simulink model "adaptive_observer_for_sin_signal_original"  (R2021b)
settings: Solver=ode4  StartTime=0.0  StopTime=simulationTime  FixedStep=0.0001  RelTol=1e-3
model workspace: external: MATLAB File D:\practice\sci\variables2n1.m (data not in the file)
values from neighbouring files (symbols this model uses):
  A = zeros(2*dimension+1 , 2*dimension+1)    [LCAD.m]
  alpha = [1,3]    [variables2n1.m]
  amp = [1;1]    [variables2n1.m]
  amp_M = [1;1]    [variables2n1.m]
  amp_M1 = 0.2    [variables2n1.m]
  bias = [0;0]    [variables2n1.m]
  bias_M = [0;0]    [variables2n1.m]
  bias_M1 = 0    [variables2n1.m]
  bigGammaZ0 = zeros(2*dimension+1, dimension)    [variables2n1.m]
  C = zeros(1, 2*dimension+1)    [LCAD.m]
  delta = C*A    [LCAD.m]    (also in stats.m = 0.05)
  dimension = 2    [variables2n1.m]
  freq = [2;3]    [variables2n1.m]
  freq_M = [1.8;3.2]    [variables2n1.m]
  freq_M1 = 20    [variables2n1.m]
  freqSwitcher = [80,150]    [variables2n1.m]
  gamma_my = 0.01    [starter3.m]
  h_my = 0.3    [starter3.m]
  initialTheta = [initialOmega(1)^2-alpha(1);     initialOmega(2)^2-alpha(2)]    [variables2n1.m]
  initialZ = [sin(phase(1)); r^2*cos(phase(1))/initialOmega(1);     sin(phase(2)); r^2*cos(phase(2))/initialOmega(2); sum(bias)]    [variables2n1.m]
  k_my = 100    [starter3.m]
  L = real((place(A',C',eigenvalues))')    [LCAD.m]
  mu = 25    [graphs.m]    (also in plot_pres4.m = 2.5; variables2n1.m = 2.5)
  noiseOrSin = 0    [variables2n1.m]
  noiseOrSwitch = 0    [variables2n1.m]
  omega1 = ones(1, length(time))*2    [graphs.m]    (also in starter3.m = 2)
  omega2 = ones(1, length(time))*3    [graphs.m]    (also in starter3.m = 3)
  omega_max = 10    [starter3.m]
  omega_min = 1    [starter3.m]
  omegaLimiter = sqrt(dimension)*maxOmega    [variables2n1.m]
  phase = [0;0]    [variables2n1.m]
  phase_M = [0;0]    [variables2n1.m]
  phase_M1 = 0    [variables2n1.m]
  r = 1.2    [variables2n1.m]
  sample_M1 = 10    [variables2n1.m]
  tau_my = 0.3    [starter3.m]
  theta0_my = [-2; 1]    [starter3.m]
  theta_real = [-c1-c2; c1*c2]    [starter3.m]
  turn_mods_on = 1    [variables2n1.m]
  zMax = 5    [variables2n1.m]
undefined symbols (not defined in the file or in its folder): G, isComplex, L1
libraries: simulink x1
(part 1 of 3)
settings Model: Creator=ASUS  LastModifiedBy=ASUS

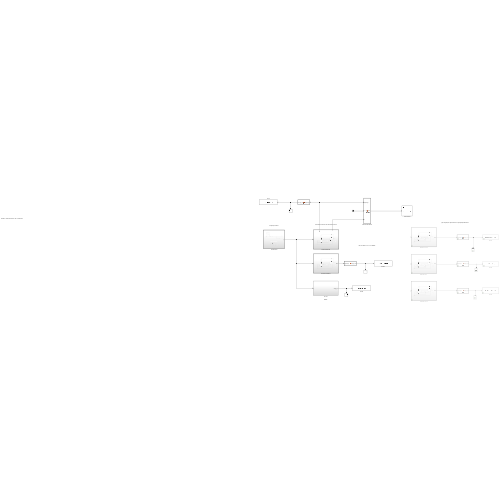
[thumbnail: Simulink's stored preview of the top-level diagram]
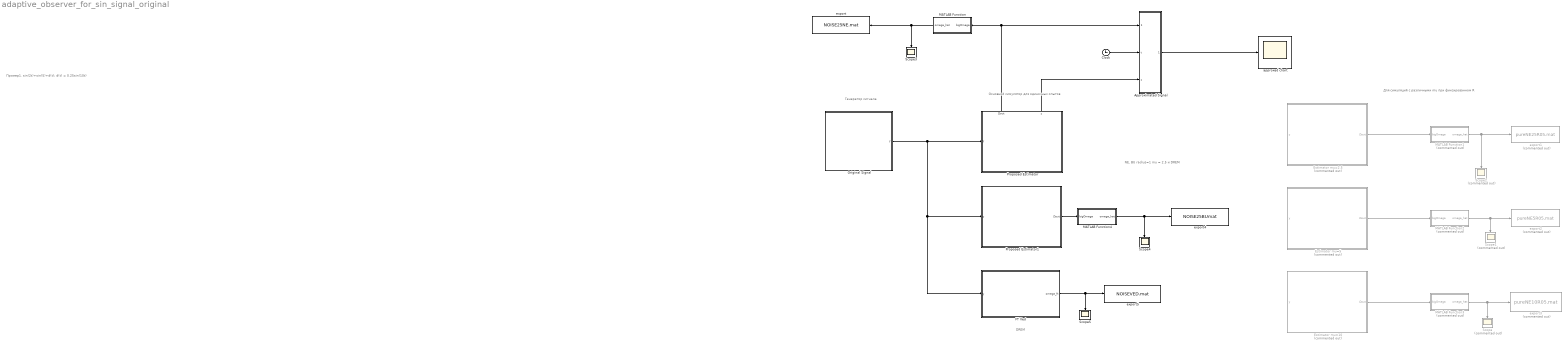
== system adaptive_observer_for_sin_signal_original ==
  note: DREM
  note: Генератор сигнала
  note: Основной симулятор для одиночных опытов
  note: Для симуляций с различными mu при фиксированном R
  note: NE, BU radius=1 mu = 2.5 и DREM
  note: Пример1. sin(2t)+sin(5)+d(t); d(t) = 0.25sin(10t)
  Approximated Signal : MATLAB Function  TreatAsAtomicUnit=on
  Clock : Clock
  Estimator mu=10 : Subsystem  Priority=2  Commented=on  TreatAsAtomicUnit=on
  Estimator mu=2.5 : Subsystem  Priority=2  Commented=on  TreatAsAtomicUnit=on
  Estimator mu=5 : Subsystem  Priority=2  Commented=on  TreatAsAtomicUnit=on
  FT Ved : Subsystem
  MATLAB Function : MATLAB Function  TreatAsAtomicUnit=on
  MATLAB Function1 : MATLAB Function  Commented=on  TreatAsAtomicUnit=on
  MATLAB Function2 : MATLAB Function  Commented=on  TreatAsAtomicUnit=on
  MATLAB Function3 : MATLAB Function  Commented=on  TreatAsAtomicUnit=on
  MATLAB Function4 : MATLAB Function  TreatAsAtomicUnit=on
  Original Signal : Subsystem  Priority=1  TreatAsAtomicUnit=on
  Proposed Estimator : Subsystem  Priority=2  TreatAsAtomicUnit=on
      settings: PortSchema="{\"entries\":[{\"content\":{\"sides\":[{\"content\":{\"connectorIds\":[\"In1\"]},\"type\":\"ConnectorPlacement.EquallySpacedRectSide\",\"uuid\":\"aaf14987-3f40-4b34-b366-ded74c88fbf6\"},{\"content\":{\"connectorIds\":[],\"side\":\"RIGHT\"},\"type\":\"ConnectorPlacement.EquallySpacedRectSide\",\"uuid\":\"c64b6003-6675-4c3e-855a-6bb89f1643de\"},{\"content\":{\"connectorIds\":[\"Out1\",\"Out2\"],\"side\":\"TOP\"},\"type\":\"ConnectorPlacement.EquallySpacedRectSide\",\"uuid\":\"73f281aa-621e-4d37-ab39-3b87d797de55\"}]},\"type\":\"ConnectorPlacement.EquallySpacedConnector\",\"uuid\":\"834767e8-0f9a-475e-a3b3-531c69e18da1\"}],\"packageUris\":[\"http://schema.mathworks.com/mf0/Connector/R2020b\"],\"version\":\"1.0\"}"
  Proposed Estimator1 : Subsystem  Priority=2  TreatAsAtomicUnit=on
  Scope : Scope  Commented=on
  Scope1 : Scope  Commented=on
  Scope2 : Scope  Commented=on
  Scope3 : Scope
  Scope4 : Scope
  Scope5 : Scope
  approxed chart : Scope
  export : ToFile  Filename=NOISE25NE.mat  MatrixName=approx_mu1
  export1 : ToFile  Commented=on  Filename=pureNE25R05.mat  MatrixName=approx_mu2_5
  export2 : ToFile  Commented=on  Filename=pureNE5R05.mat  MatrixName=approx_mu_5
  export3 : ToFile  Commented=on  Filename=pureNE10R05.mat  MatrixName=approx_mu_10
  export4 : ToFile  Filename=NOISE25BUmat  MatrixName=approx_mu1
  export5 : ToFile  Filename=NOISEVED.mat  MatrixName=approx_mu1
  wires:
  Approximated Signal/1(sgn_value) -> approxed chart/1
  Clock/1 -> Approximated Signal/2(t)
  Original Signal/1(y) -> FT Ved/1(y), Proposed Estimator1/1(y), Proposed Estimator/1(y)
  Proposed Estimator/2(z) -> Approximated Signal/3(z)
  Proposed Estimator/1(Ωout) -> Approximated Signal/1(bigOmega), MATLAB Function/1(bigOmega)
  MATLAB Function/1(omega_hat) -> export/1, Scope3/1
  MATLAB Function1/1(omega_hat) -> export1/1, Scope2/1
  Estimator mu=2.5/1(Ωout) -> MATLAB Function1/1(bigOmega)
  Estimator mu=5/1(Ωout) -> MATLAB Function2/1(bigOmega)
  MATLAB Function2/1(omega_hat) -> Scope1/1, export2/1
  Estimator mu=10/1(Ωout) -> MATLAB Function3/1(bigOmega)
  MATLAB Function3/1(omega_hat) -> export3/1, Scope/1
  Proposed Estimator1/1(Ωout) -> MATLAB Function4/1(bigOmega)
  FT Ved/1(omega_ft) -> Scope5/1, export5/1
  MATLAB Function4/1(omega_hat) -> Scope4/1, export4/1

== system adaptive_observer_for_sin_signal_original/Estimator mu=10 ==
  note: Оценщик Ω
  note: Оценщик Φ
  note: Оценщик z
  y : Inport
  Frequencies estimator : Subsystem
      settings: PortSchema="{\"entries\":[{\"content\":{\"sides\":[{\"content\":{\"connectorIds\":[\"In1\",\"In2\"]},\"type\":\"ConnectorPlacement.EquallySpacedRectSide\",\"uuid\":\"56415c13-d553-4f88-94d3-75bcdc800e4b\"},{\"content\":{\"connectorIds\":[\"Out1\"],\"side\":\"RIGHT\"},\"type\":\"ConnectorPlacement.EquallySpacedRectSide\",\"uuid\":\"a1bdd2d2-4e49-40cb-b0b7-1df5316e4510\"},{\"content\":{\"connectorIds\":[\"In3\"],\"side\":\"TOP\"},\"type\":\"ConnectorPlacement.EquallySpacedRectSide\",\"uuid\":\"59b6ba3d-4a55-43e8-9b14-0d873cc3c9ca\"},{\"content\":{\"connectorIds\":[\"In4\",\"In5\"],\"side\":\"BOTTOM\"},\"type\":\"ConnectorPlacement.EquallySpacedRectSide\",\"uuid\":\"70a04625-4f15-4458-8acb-2ccaa963f28c\"}]},\"type\":\"ConnectorPlacement.EquallySpacedConnector\",\"uuid\":\"fdf2e112-ecff-41aa-a5cb-d527a9dd51a8\"}],\"packageUris\":[\"http://schema.mathworks.com/mf0/Connector/R2020b\"],\"version\":\"1.0\"}"
  Subsystem : Subsystem  Priority=6  TreatAsAtomicUnit=on
  Subsystem1 : Subsystem  Commented=on
  z' : Subsystem  Priority=7  TreatAsAtomicUnit=on
      settings: PortSchema="{\"entries\":[{\"content\":{\"sides\":[{\"content\":{\"connectorIds\":[\"In1\",\"In2\"]},\"type\":\"ConnectorPlacement.EquallySpacedRectSide\",\"uuid\":\"ef8cffdc-1e6f-42c0-8cb3-bf318ca182f8\"},{\"content\":{\"connectorIds\":[\"Out1\"],\"side\":\"RIGHT\"},\"type\":\"ConnectorPlacement.EquallySpacedRectSide\",\"uuid\":\"a9c7e5b7-281a-47aa-808a-eb2877f3eee0\"},{\"content\":{\"connectorIds\":[\"In3\"],\"side\":\"TOP\"},\"type\":\"ConnectorPlacement.EquallySpacedRectSide\",\"uuid\":\"7bb4f6b5-7deb-4e08-9b2d-b96cfbb2c85e\"},{\"content\":{\"connectorIds\":[\"In4\"],\"side\":\"BOTTOM\"},\"type\":\"ConnectorPlacement.EquallySpacedRectSide\",\"uuid\":\"fa3b2d15-5a15-4cf8-893e-51642802107c\"}]},\"type\":\"ConnectorPlacement.EquallySpacedConnector\",\"uuid\":\"64fccc24-315d-40ff-920f-bd434d551c1a\"}],\"packageUris\":[\"http://schema.mathworks.com/mf0/Connector/R2020b\"],\"version\":\"1.0\"}"
  Г(z) : MATLAB Function  Priority=2  TreatAsAtomicUnit=on
  "∫Z " : Integrator  Priority=1  InitialCondition=initialZ
  Ωout : Outport
  wires:
  z'/1(z') -> "∫Z "/1, Frequencies estimator/2(ż)
  Г(z)/1(bigGammaZ) -> z'/2(Г(z))
  Frequencies estimator/1(Ω out) -> Subsystem/1(Ω), Frequencies estimator/3(Ω in), Ωout/1
  y/1 -> Frequencies estimator/5(y), z'/1(y)
  Subsystem/1(Ф) -> z'/3(Ф), Frequencies estimator/1(Ф)
  "∫Z "/1 -> Frequencies estimator/4(z), Г(z)/1(z), z'/4(z)

== system adaptive_observer_for_sin_signal_original/Estimator mu=2.5 ==
  note: Оценщик Ω
  note: Оценщик Φ
  note: Оценщик z
  y : Inport
  Frequencies estimator : Subsystem
      settings: PortSchema="{\"entries\":[{\"content\":{\"sides\":[{\"content\":{\"connectorIds\":[\"In1\",\"In2\"]},\"type\":\"ConnectorPlacement.EquallySpacedRectSide\",\"uuid\":\"56415c13-d553-4f88-94d3-75bcdc800e4b\"},{\"content\":{\"connectorIds\":[\"Out1\"],\"side\":\"RIGHT\"},\"type\":\"ConnectorPlacement.EquallySpacedRectSide\",\"uuid\":\"a1bdd2d2-4e49-40cb-b0b7-1df5316e4510\"},{\"content\":{\"connectorIds\":[\"In3\"],\"side\":\"TOP\"},\"type\":\"ConnectorPlacement.EquallySpacedRectSide\",\"uuid\":\"59b6ba3d-4a55-43e8-9b14-0d873cc3c9ca\"},{\"content\":{\"connectorIds\":[\"In4\",\"In5\"],\"side\":\"BOTTOM\"},\"type\":\"ConnectorPlacement.EquallySpacedRectSide\",\"uuid\":\"70a04625-4f15-4458-8acb-2ccaa963f28c\"}]},\"type\":\"ConnectorPlacement.EquallySpacedConnector\",\"uuid\":\"fdf2e112-ecff-41aa-a5cb-d527a9dd51a8\"}],\"packageUris\":[\"http://schema.mathworks.com/mf0/Connector/R2020b\"],\"version\":\"1.0\"}"
  Subsystem : Subsystem  Priority=6  TreatAsAtomicUnit=on
  Subsystem1 : Subsystem  Commented=on
  z' : Subsystem  Priority=7  TreatAsAtomicUnit=on
      settings: PortSchema="{\"entries\":[{\"content\":{\"sides\":[{\"content\":{\"connectorIds\":[\"In1\",\"In2\"]},\"type\":\"ConnectorPlacement.EquallySpacedRectSide\",\"uuid\":\"ef8cffdc-1e6f-42c0-8cb3-bf318ca182f8\"},{\"content\":{\"connectorIds\":[\"Out1\"],\"side\":\"RIGHT\"},\"type\":\"ConnectorPlacement.EquallySpacedRectSide\",\"uuid\":\"a9c7e5b7-281a-47aa-808a-eb2877f3eee0\"},{\"content\":{\"connectorIds\":[\"In3\"],\"side\":\"TOP\"},\"type\":\"ConnectorPlacement.EquallySpacedRectSide\",\"uuid\":\"7bb4f6b5-7deb-4e08-9b2d-b96cfbb2c85e\"},{\"content\":{\"connectorIds\":[\"In4\"],\"side\":\"BOTTOM\"},\"type\":\"ConnectorPlacement.EquallySpacedRectSide\",\"uuid\":\"fa3b2d15-5a15-4cf8-893e-51642802107c\"}]},\"type\":\"ConnectorPlacement.EquallySpacedConnector\",\"uuid\":\"64fccc24-315d-40ff-920f-bd434d551c1a\"}],\"packageUris\":[\"http://schema.mathworks.com/mf0/Connector/R2020b\"],\"version\":\"1.0\"}"
  Г(z) : MATLAB Function  Priority=2  TreatAsAtomicUnit=on
  "∫Z " : Integrator  Priority=1  InitialCondition=initialZ
  Ωout : Outport
  wires:
  z'/1(z') -> "∫Z "/1, Frequencies estimator/2(ż)
  Г(z)/1(bigGammaZ) -> z'/2(Г(z))
  Frequencies estimator/1(Ω out) -> Subsystem/1(Ω), Frequencies estimator/3(Ω in), Ωout/1
  y/1 -> Frequencies estimator/5(y), z'/1(y)
  Subsystem/1(Ф) -> z'/3(Ф), Frequencies estimator/1(Ф)
  "∫Z "/1 -> Frequencies estimator/4(z), Г(z)/1(z), z'/4(z)

== system adaptive_observer_for_sin_signal_original/Estimator mu=5 ==
  note: Оценщик Ω
  note: Оценщик Φ
  note: Оценщик z
  y : Inport
  Frequencies estimator : Subsystem
      settings: PortSchema="{\"entries\":[{\"content\":{\"sides\":[{\"content\":{\"connectorIds\":[\"In1\",\"In2\"]},\"type\":\"ConnectorPlacement.EquallySpacedRectSide\",\"uuid\":\"56415c13-d553-4f88-94d3-75bcdc800e4b\"},{\"content\":{\"connectorIds\":[\"Out1\"],\"side\":\"RIGHT\"},\"type\":\"ConnectorPlacement.EquallySpacedRectSide\",\"uuid\":\"a1bdd2d2-4e49-40cb-b0b7-1df5316e4510\"},{\"content\":{\"connectorIds\":[\"In3\"],\"side\":\"TOP\"},\"type\":\"ConnectorPlacement.EquallySpacedRectSide\",\"uuid\":\"59b6ba3d-4a55-43e8-9b14-0d873cc3c9ca\"},{\"content\":{\"connectorIds\":[\"In4\",\"In5\"],\"side\":\"BOTTOM\"},\"type\":\"ConnectorPlacement.EquallySpacedRectSide\",\"uuid\":\"70a04625-4f15-4458-8acb-2ccaa963f28c\"}]},\"type\":\"ConnectorPlacement.EquallySpacedConnector\",\"uuid\":\"fdf2e112-ecff-41aa-a5cb-d527a9dd51a8\"}],\"packageUris\":[\"http://schema.mathworks.com/mf0/Connector/R2020b\"],\"version\":\"1.0\"}"
  Subsystem : Subsystem  Priority=6  TreatAsAtomicUnit=on
  Subsystem1 : Subsystem  Commented=on
  z' : Subsystem  Priority=7  TreatAsAtomicUnit=on
      settings: PortSchema="{\"entries\":[{\"content\":{\"sides\":[{\"content\":{\"connectorIds\":[\"In1\",\"In2\"]},\"type\":\"ConnectorPlacement.EquallySpacedRectSide\",\"uuid\":\"ef8cffdc-1e6f-42c0-8cb3-bf318ca182f8\"},{\"content\":{\"connectorIds\":[\"Out1\"],\"side\":\"RIGHT\"},\"type\":\"ConnectorPlacement.EquallySpacedRectSide\",\"uuid\":\"a9c7e5b7-281a-47aa-808a-eb2877f3eee0\"},{\"content\":{\"connectorIds\":[\"In3\"],\"side\":\"TOP\"},\"type\":\"ConnectorPlacement.EquallySpacedRectSide\",\"uuid\":\"7bb4f6b5-7deb-4e08-9b2d-b96cfbb2c85e\"},{\"content\":{\"connectorIds\":[\"In4\"],\"side\":\"BOTTOM\"},\"type\":\"ConnectorPlacement.EquallySpacedRectSide\",\"uuid\":\"fa3b2d15-5a15-4cf8-893e-51642802107c\"}]},\"type\":\"ConnectorPlacement.EquallySpacedConnector\",\"uuid\":\"64fccc24-315d-40ff-920f-bd434d551c1a\"}],\"packageUris\":[\"http://schema.mathworks.com/mf0/Connector/R2020b\"],\"version\":\"1.0\"}"
  Г(z) : MATLAB Function  Priority=2  TreatAsAtomicUnit=on
  "∫Z " : Integrator  Priority=1  InitialCondition=initialZ
  Ωout : Outport
  wires:
  z'/1(z') -> "∫Z "/1, Frequencies estimator/2(ż)
  Г(z)/1(bigGammaZ) -> z'/2(Г(z))
  Frequencies estimator/1(Ω out) -> Subsystem/1(Ω), Frequencies estimator/3(Ω in), Ωout/1
  y/1 -> Frequencies estimator/5(y), z'/1(y)
  Subsystem/1(Ф) -> z'/3(Ф), Frequencies estimator/1(Ф)
  "∫Z "/1 -> Frequencies estimator/4(z), Г(z)/1(z), z'/4(z)

== system adaptive_observer_for_sin_signal_original/FT Ved ==
  y : Inport
  Constant : Constant  Value=[omega1; omega2]
  DREM : Subsystem
  Gradient1 : Subsystem
  MATLAB Function2 : MATLAB Function  TreatAsAtomicUnit=on
  Regression model : Subsystem
  Scope : Scope
  Scope1 : Scope  NumInputPorts=2
  omega_ft : Outport  VectorParamsAs1DForOutWhenUnconnected=off
  wires:
  Regression model/1(psi) -> DREM/1(psi)
  DREM/1(PSI) -> Gradient1/1(PSI)
  DREM/2(PHI) -> Gradient1/2(PHI)
  Regression model/3(theta) -> DREM/3(theta)
  y/1 -> Regression model/1(y)
  Constant/1 -> Scope1/2
  Regression model/2(phi) -> DREM/2(phi)
  MATLAB Function2/1(omega_hat) -> omega_ft/1, Scope1/1
  Gradient1/1(theta_hat_ft) -> MATLAB Function2/1(theta_hat)
  MATLAB Function2/2(Q) -> Scope/1

== system adaptive_observer_for_sin_signal_original/Original Signal ==
  note: Настроить по формулам чистого осциллятора. Применять для уточнения оценок zMax. Домноженный на C даёт сигнал y.
  note: Переключатель сигнала. Включает внешние воздействия при turn_mods_on=1
  Clock : Clock  Commented=on
  Comparsion Osc : Scope
  Gain : Gain  Commented=on  Gain=G  Multiplication=Matrix(K*u)
  Gain1 : Gain  Commented=on  Gain=C  Multiplication=Matrix(K*u)
  Gz : Scope  Commented=on
  Integrator : Integrator  Commented=on  InitialCondition=[0;(r^2)/2;0;(r^2)/3;0]
  MATLAB Function : MATLAB Function  Commented=on  TreatAsAtomicUnit=on
  Memory : Memory  Commented=on
  Source Signal : Subsystem
  Switcher : Switch  Criteria=u2 > Threshold  Threshold=freqSwitcher(1)
  modifier : Subsystem
  mods enabler : Subsystem
  z Pure : Scope  Commented=on
  zMax : Display  Commented=on
  y : Outport
  wires:
  Gain/1 -> Gz/1, Integrator/1
  Integrator/1 -> MATLAB Function/1(z), z Pure/1, Gain1/1, Gain/1
  MATLAB Function/1(zSup) -> Memory/1, zMax/1
  Clock/1 -> MATLAB Function/2(t)
  Memory/1 -> MATLAB Function/3(zPrev)
  mods enabler/1(on_off) -> Switcher/2
  modifier/1(y_mod) -> Switcher/1
  Source Signal/1(y) -> modifier/1(y), Switcher/3
  Switcher/1 -> y/1, Comparsion Osc/1
  Gain1/1 -> ?

== system adaptive_observer_for_sin_signal_original/Proposed Estimator ==
  note: Оценщик Ω
  note: Оценщик Φ
  note: Оценщик z
  y : Inport
  Frequencies estimator : Subsystem
      settings: PortSchema="{\"entries\":[{\"content\":{\"sides\":[{\"content\":{\"connectorIds\":[\"In1\",\"In2\"]},\"type\":\"ConnectorPlacement.EquallySpacedRectSide\",\"uuid\":\"56415c13-d553-4f88-94d3-75bcdc800e4b\"},{\"content\":{\"connectorIds\":[\"Out1\"],\"side\":\"RIGHT\"},\"type\":\"ConnectorPlacement.EquallySpacedRectSide\",\"uuid\":\"a1bdd2d2-4e49-40cb-b0b7-1df5316e4510\"},{\"content\":{\"connectorIds\":[\"In3\"],\"side\":\"TOP\"},\"type\":\"ConnectorPlacement.EquallySpacedRectSide\",\"uuid\":\"59b6ba3d-4a55-43e8-9b14-0d873cc3c9ca\"},{\"content\":{\"connectorIds\":[\"In4\",\"In5\"],\"side\":\"BOTTOM\"},\"type\":\"ConnectorPlacement.EquallySpacedRectSide\",\"uuid\":\"70a04625-4f15-4458-8acb-2ccaa963f28c\"}]},\"type\":\"ConnectorPlacement.EquallySpacedConnector\",\"uuid\":\"fdf2e112-ecff-41aa-a5cb-d527a9dd51a8\"}],\"packageUris\":[\"http://schema.mathworks.com/mf0/Connector/R2020b\"],\"version\":\"1.0\"}"
  Subsystem : Subsystem  Priority=6  TreatAsAtomicUnit=on
  Subsystem1 : Subsystem  Commented=on
  z' : Subsystem  Priority=7  TreatAsAtomicUnit=on
      settings: PortSchema="{\"entries\":[{\"content\":{\"sides\":[{\"content\":{\"connectorIds\":[\"In1\",\"In2\"]},\"type\":\"ConnectorPlacement.EquallySpacedRectSide\",\"uuid\":\"ef8cffdc-1e6f-42c0-8cb3-bf318ca182f8\"},{\"content\":{\"connectorIds\":[\"Out1\"],\"side\":\"RIGHT\"},\"type\":\"ConnectorPlacement.EquallySpacedRectSide\",\"uuid\":\"a9c7e5b7-281a-47aa-808a-eb2877f3eee0\"},{\"content\":{\"connectorIds\":[\"In3\"],\"side\":\"TOP\"},\"type\":\"ConnectorPlacement.EquallySpacedRectSide\",\"uuid\":\"7bb4f6b5-7deb-4e08-9b2d-b96cfbb2c85e\"},{\"content\":{\"connectorIds\":[\"In4\"],\"side\":\"BOTTOM\"},\"type\":\"ConnectorPlacement.EquallySpacedRectSide\",\"uuid\":\"fa3b2d15-5a15-4cf8-893e-51642802107c\"}]},\"type\":\"ConnectorPlacement.EquallySpacedConnector\",\"uuid\":\"64fccc24-315d-40ff-920f-bd434d551c1a\"}],\"packageUris\":[\"http://schema.mathworks.com/mf0/Connector/R2020b\"],\"version\":\"1.0\"}"
  Г(z) : MATLAB Function  Priority=2  TreatAsAtomicUnit=on
  "∫Z " : Integrator  Priority=1  InitialCondition=initialZ
  Ωout : Outport
  z : Outport  Port=2
  wires:
  z'/1(z') -> "∫Z "/1, Frequencies estimator/2(ż)
  Г(z)/1(bigGammaZ) -> z'/2(Г(z))
  Frequencies estimator/1(Ω out) -> Subsystem/1(Ω), Frequencies estimator/3(Ω in), Ωout/1
  y/1 -> Frequencies estimator/5(y), z'/1(y)
  Subsystem/1(Ф) -> z'/3(Ф), Frequencies estimator/1(Ф)
  "∫Z "/1 -> Frequencies estimator/4(z), z/1, Г(z)/1(z), z'/4(z)

== system adaptive_observer_for_sin_signal_original/Proposed Estimator1 ==
  note: Оценщик Ω
  note: Оценщик Φ
  note: Оценщик z
  y : Inport
  Frequencies estimator : Subsystem
      settings: PortSchema="{\"entries\":[{\"content\":{\"sides\":[{\"content\":{\"connectorIds\":[\"In1\",\"In2\"]},\"type\":\"ConnectorPlacement.EquallySpacedRectSide\",\"uuid\":\"56415c13-d553-4f88-94d3-75bcdc800e4b\"},{\"content\":{\"connectorIds\":[\"Out1\"],\"side\":\"RIGHT\"},\"type\":\"ConnectorPlacement.EquallySpacedRectSide\",\"uuid\":\"a1bdd2d2-4e49-40cb-b0b7-1df5316e4510\"},{\"content\":{\"connectorIds\":[\"In3\"],\"side\":\"TOP\"},\"type\":\"ConnectorPlacement.EquallySpacedRectSide\",\"uuid\":\"59b6ba3d-4a55-43e8-9b14-0d873cc3c9ca\"},{\"content\":{\"connectorIds\":[\"In4\",\"In5\"],\"side\":\"BOTTOM\"},\"type\":\"ConnectorPlacement.EquallySpacedRectSide\",\"uuid\":\"70a04625-4f15-4458-8acb-2ccaa963f28c\"}]},\"type\":\"ConnectorPlacement.EquallySpacedConnector\",\"uuid\":\"fdf2e112-ecff-41aa-a5cb-d527a9dd51a8\"}],\"packageUris\":[\"http://schema.mathworks.com/mf0/Connector/R2020b\"],\"version\":\"1.0\"}"
  Subsystem : Subsystem  Priority=6  TreatAsAtomicUnit=on
  Subsystem1 : Subsystem  Commented=on
  z' : Subsystem  Priority=7  TreatAsAtomicUnit=on
      settings: PortSchema="{\"entries\":[{\"content\":{\"sides\":[{\"content\":{\"connectorIds\":[\"In1\",\"In2\"]},\"type\":\"ConnectorPlacement.EquallySpacedRectSide\",\"uuid\":\"ef8cffdc-1e6f-42c0-8cb3-bf318ca182f8\"},{\"content\":{\"connectorIds\":[\"Out1\"],\"side\":\"RIGHT\"},\"type\":\"ConnectorPlacement.EquallySpacedRectSide\",\"uuid\":\"a9c7e5b7-281a-47aa-808a-eb2877f3eee0\"},{\"content\":{\"connectorIds\":[\"In3\"],\"side\":\"TOP\"},\"type\":\"ConnectorPlacement.EquallySpacedRectSide\",\"uuid\":\"7bb4f6b5-7deb-4e08-9b2d-b96cfbb2c85e\"},{\"content\":{\"connectorIds\":[\"In4\"],\"side\":\"BOTTOM\"},\"type\":\"ConnectorPlacement.EquallySpacedRectSide\",\"uuid\":\"fa3b2d15-5a15-4cf8-893e-51642802107c\"}]},\"type\":\"ConnectorPlacement.EquallySpacedConnector\",\"uuid\":\"64fccc24-315d-40ff-920f-bd434d551c1a\"}],\"packageUris\":[\"http://schema.mathworks.com/mf0/Connector/R2020b\"],\"version\":\"1.0\"}"
  Г(z) : MATLAB Function  Priority=2  TreatAsAtomicUnit=on
  "∫Z " : Integrator  Priority=1  InitialCondition=initialZ
  Ωout : Outport
  wires:
  z'/1(z') -> "∫Z "/1, Frequencies estimator/2(ż)
  Г(z)/1(bigGammaZ) -> z'/2(Г(z))
  Frequencies estimator/1(Ω out) -> Subsystem/1(Ω), Frequencies estimator/3(Ω in), Ωout/1
  y/1 -> Frequencies estimator/5(y), z'/1(y)
  Subsystem/1(Ф) -> z'/3(Ф), Frequencies estimator/1(Ф)
  "∫Z "/1 -> Frequencies estimator/4(z), Г(z)/1(z), z'/4(z)

== system adaptive_observer_for_sin_signal_original/Estimator mu=10/Frequencies estimator ==
  Ф : Inport
  ż : Inport  Port=2
  Ω in : Inport  Port=3
  z : Inport  Port=4
  y : Inport  Port=5
  Fc : Subsystem  Priority=8  TreatAsAtomicUnit=on
      settings: PortSchema="{\"entries\":[{\"content\":{\"sides\":[{\"content\":{\"connectorIds\":[\"In1\",\"In2\",\"In3\"]},\"type\":\"ConnectorPlacement.EquallySpacedRectSide\",\"uuid\":\"ef8cffdc-1e6f-42c0-8cb3-bf318ca182f8\"},{\"content\":{\"connectorIds\":[\"Out1\"],\"side\":\"RIGHT\"},\"type\":\"ConnectorPlacement.EquallySpacedRectSide\",\"uuid\":\"a9c7e5b7-281a-47aa-808a-eb2877f3eee0\"},{\"content\":{\"connectorIds\":[\"In4\"],\"side\":\"TOP\"},\"type\":\"ConnectorPlacement.EquallySpacedRectSide\",\"uuid\":\"7bb4f6b5-7deb-4e08-9b2d-b96cfbb2c85e\"},{\"content\":{\"connectorIds\":[],\"side\":\"BOTTOM\"},\"type\":\"ConnectorPlacement.EquallySpacedRectSide\",\"uuid\":\"d628d464-6f95-4c60-8de5-a9188665a8a2\"}]},\"type\":\"ConnectorPlacement.EquallySpacedConnector\",\"uuid\":\"64fccc24-315d-40ff-920f-bd434d551c1a\"}],\"packageUris\":[\"http://schema.mathworks.com/mf0/Connector/R2020b\"],\"version\":\"1.0\"}"
  Fu : Subsystem  Priority=9  TreatAsAtomicUnit=on
      settings: PortSchema="{\"entries\":[{\"content\":{\"sides\":[{\"content\":{\"connectorIds\":[\"In1\",\"In2\"]},\"type\":\"ConnectorPlacement.EquallySpacedRectSide\",\"uuid\":\"56415c13-d553-4f88-94d3-75bcdc800e4b\"},{\"content\":{\"connectorIds\":[\"Out1\"],\"side\":\"RIGHT\"},\"type\":\"ConnectorPlacement.EquallySpacedRectSide\",\"uuid\":\"a1bdd2d2-4e49-40cb-b0b7-1df5316e4510\"},{\"content\":{\"connectorIds\":[\"In3\"],\"side\":\"TOP\"},\"type\":\"ConnectorPlacement.EquallySpacedRectSide\",\"uuid\":\"59b6ba3d-4a55-43e8-9b14-0d873cc3c9ca\"},{\"content\":{\"connectorIds\":[\"In4\",\"In5\"],\"side\":\"BOTTOM\"},\"type\":\"ConnectorPlacement.EquallySpacedRectSide\",\"uuid\":\"cb3db39e-f643-4fe7-a27f-76e86359c78d\"}]},\"type\":\"ConnectorPlacement.EquallySpacedConnector\",\"uuid\":\"fdf2e112-ecff-41aa-a5cb-d527a9dd51a8\"}],\"packageUris\":[\"http://schema.mathworks.com/mf0/Connector/R2020b\"],\"version\":\"1.0\"}"
  Ω : Subsystem  Priority=5  TreatAsAtomicUnit=on
      settings: PortSchema="{\"entries\":[{\"content\":{\"sides\":[{\"content\":{\"connectorIds\":[\"In1\",\"In2\"]},\"type\":\"ConnectorPlacement.EquallySpacedRectSide\",\"uuid\":\"0172ca52-64e8-432c-895c-e5829558e278\"},{\"content\":{\"connectorIds\":[\"Out1\"],\"side\":\"RIGHT\"},\"type\":\"ConnectorPlacement.EquallySpacedRectSide\",\"uuid\":\"c83f4e01-5d94-498a-a9de-b4a302d500ab\"},{\"content\":{\"connectorIds\":[\"In3\"],\"side\":\"TOP\"},\"type\":\"ConnectorPlacement.EquallySpacedRectSide\",\"uuid\":\"3a6496e3-470c-4361-9f8f-cd28e1556398\"}]},\"type\":\"ConnectorPlacement.EquallySpacedConnector\",\"uuid\":\"b738ec8a-20ee-4a0a-8362-4988f331d970\"}],\"packageUris\":[\"http://schema.mathworks.com/mf0/Connector/R2020b\"],\"version\":\"1.0\"}"
  θ' : Subsystem  Priority=10  TreatAsAtomicUnit=on
      settings: PortSchema="{\"entries\":[{\"content\":{\"sides\":[{\"content\":{\"connectorIds\":[\"In1\"]},\"type\":\"ConnectorPlacement.EquallySpacedRectSide\",\"uuid\":\"9184f415-d771-478b-8114-38f854f6aad6\"},{\"content\":{\"connectorIds\":[\"Out1\"],\"side\":\"RIGHT\"},\"type\":\"ConnectorPlacement.EquallySpacedRectSide\",\"uuid\":\"399c2935-e635-4d1c-9ba7-451eea57bae3\"},{\"content\":{\"connectorIds\":[\"In2\"],\"side\":\"TOP\"},\"type\":\"ConnectorPlacement.EquallySpacedRectSide\",\"uuid\":\"bdc6ec05-8dca-4996-ba70-702aa29fd179\"}]},\"type\":\"ConnectorPlacement.EquallySpacedConnector\",\"uuid\":\"fa68c3f3-8285-4ee8-b99d-908dba81143c\"}],\"packageUris\":[\"http://schema.mathworks.com/mf0/Connector/R2020b\"],\"version\":\"1.0\"}"
  г(z) : Selector  InputPortWidth=2*dimension+1  IndexOptions=Index vector (dialog)  Indices=2:2:2*dimension  OutputSizes=1
  "∫θ " : Integrator  Priority=3  InitialCondition=initialTheta
  Ω out : Outport
  wires:
  Ф/1 -> Fu/1(Ф), Fc/3(Ф)
  y/1 -> Ω/2(y), Fu/5(y)
  z/1 -> г(z)/1, Fu/2(z), Fc/1(z)
  г(z)/1 -> Fc/4(Г(z)), Ω/3(г(z)), Fu/4(г(z))
  Ω in/1 -> Fc/2(Ω)
  ż/1 -> Fu/3(ż)
  "∫θ "/1 -> Ω/1(θ)
  Ω/1(Ω) -> Ω out/1
  Fc/1(Fc) -> θ'/2(Fc)
  Fu/1(Fu) -> θ'/1(Fu)
  θ'/1(θ') -> "∫θ "/1

== system adaptive_observer_for_sin_signal_original/Estimator mu=10/Subsystem ==
  Ω : Inport
  Constant1 : Constant  Value=r^2
  Divide : Product  Inputs=*/
  Gain1 : Gain  Gain=r^2
  Transpose{,1..3} (4 alike) : Math  Operator=transpose  SaturateOnIntegerOverflow=on
  Λ : Constant  Value=alpha
  Ω-Λ : Sum  Inputs=+-
  Ф : Outport
  wires:
  Divide/1 -> Ω-Λ/1
  Ω-Λ/1 -> Transpose1/1
  Ω/1 -> Divide/1
  Constant1/1 -> Divide/2
  Gain1/1 -> Transpose2/1
  Λ/1 -> Transpose/1
  Transpose/1 -> Gain1/1
  Transpose2/1 -> Ω-Λ/2
  Transpose1/1 -> Transpose3/1
  Transpose3/1 -> Ф/1

== system adaptive_observer_for_sin_signal_original/Estimator mu=10/Subsystem1 ==
  u : Inport
  Complex to Real-Imag : ComplexToRealImag
  MATLAB Function : MATLAB Function  TreatAsAtomicUnit=on
  Real-Imag to Complex : RealImagToComplex
  Switcher : Switch  Criteria=u2 ~= 0  Threshold=freqSwitcher(1)
  isComplex : Constant  Value=isComplex
  "∫Z " : Integrator  Priority=1  InitialCondition=real(initialZ)
  ∫Z 1 : Integrator  Priority=1  InitialCondition=imag(initialZ)
  Out1 : Outport
  wires:
  isComplex/1 -> Switcher/2
  u/1 -> MATLAB Function/1(zPrime), Complex to Real-Imag/1
  "∫Z "/1 -> Real-Imag to Complex/1, Switcher/1
  Switcher/1 -> Out1/1
  Complex to Real-Imag/1 -> "∫Z "/1
  Complex to Real-Imag/2 -> ∫Z 1/1
  ∫Z 1/1 -> Real-Imag to Complex/2
  Real-Imag to Complex/1 -> Switcher/3

== system adaptive_observer_for_sin_signal_original/Estimator mu=10/z' ==
  y : Inport
  Г(z) : Inport  Port=2
  Ф : Inport  Port=3
  z : Inport  Port=4
  Minus : Sum  Inputs=+-
  Product : Product  Multiplication=Matrix(*)
  S(z) : Subsystem
  Subsystem : Subsystem
  z' : Outport
  wires:
  z/1 -> Subsystem/4(z), S(z)/2(z)
  Minus/1 -> z'/1
  S(z)/1(S) -> Product/1
  Product/1 -> Minus/2
  Subsystem/1(zPreDot) -> Minus/1, Product/2, S(z)/1(zPreDot)
  Г(z)/1 -> Subsystem/1(bigGamma)
  Ф/1 -> Subsystem/2(PHI)
  y/1 -> Subsystem/3(y)

== system adaptive_observer_for_sin_signal_original/Estimator mu=2.5/Frequencies estimator ==
  Ф : Inport
  ż : Inport  Port=2
  Ω in : Inport  Port=3
  z : Inport  Port=4
  y : Inport  Port=5
  Fc : Subsystem  Priority=8  TreatAsAtomicUnit=on
      settings: PortSchema="{\"entries\":[{\"content\":{\"sides\":[{\"content\":{\"connectorIds\":[\"In1\",\"In2\",\"In3\"]},\"type\":\"ConnectorPlacement.EquallySpacedRectSide\",\"uuid\":\"ef8cffdc-1e6f-42c0-8cb3-bf318ca182f8\"},{\"content\":{\"connectorIds\":[\"Out1\"],\"side\":\"RIGHT\"},\"type\":\"ConnectorPlacement.EquallySpacedRectSide\",\"uuid\":\"a9c7e5b7-281a-47aa-808a-eb2877f3eee0\"},{\"content\":{\"connectorIds\":[\"In4\"],\"side\":\"TOP\"},\"type\":\"ConnectorPlacement.EquallySpacedRectSide\",\"uuid\":\"7bb4f6b5-7deb-4e08-9b2d-b96cfbb2c85e\"},{\"content\":{\"connectorIds\":[],\"side\":\"BOTTOM\"},\"type\":\"ConnectorPlacement.EquallySpacedRectSide\",\"uuid\":\"d628d464-6f95-4c60-8de5-a9188665a8a2\"}]},\"type\":\"ConnectorPlacement.EquallySpacedConnector\",\"uuid\":\"64fccc24-315d-40ff-920f-bd434d551c1a\"}],\"packageUris\":[\"http://schema.mathworks.com/mf0/Connector/R2020b\"],\"version\":\"1.0\"}"
  Fu : Subsystem  Priority=9  TreatAsAtomicUnit=on
      settings: PortSchema="{\"entries\":[{\"content\":{\"sides\":[{\"content\":{\"connectorIds\":[\"In1\",\"In2\"]},\"type\":\"ConnectorPlacement.EquallySpacedRectSide\",\"uuid\":\"56415c13-d553-4f88-94d3-75bcdc800e4b\"},{\"content\":{\"connectorIds\":[\"Out1\"],\"side\":\"RIGHT\"},\"type\":\"ConnectorPlacement.EquallySpacedRectSide\",\"uuid\":\"a1bdd2d2-4e49-40cb-b0b7-1df5316e4510\"},{\"content\":{\"connectorIds\":[\"In3\"],\"side\":\"TOP\"},\"type\":\"ConnectorPlacement.EquallySpacedRectSide\",\"uuid\":\"59b6ba3d-4a55-43e8-9b14-0d873cc3c9ca\"},{\"content\":{\"connectorIds\":[\"In4\",\"In5\"],\"side\":\"BOTTOM\"},\"type\":\"ConnectorPlacement.EquallySpacedRectSide\",\"uuid\":\"cb3db39e-f643-4fe7-a27f-76e86359c78d\"}]},\"type\":\"ConnectorPlacement.EquallySpacedConnector\",\"uuid\":\"fdf2e112-ecff-41aa-a5cb-d527a9dd51a8\"}],\"packageUris\":[\"http://schema.mathworks.com/mf0/Connector/R2020b\"],\"version\":\"1.0\"}"
  Ω : Subsystem  Priority=5  TreatAsAtomicUnit=on
      settings: PortSchema="{\"entries\":[{\"content\":{\"sides\":[{\"content\":{\"connectorIds\":[\"In1\",\"In2\"]},\"type\":\"ConnectorPlacement.EquallySpacedRectSide\",\"uuid\":\"0172ca52-64e8-432c-895c-e5829558e278\"},{\"content\":{\"connectorIds\":[\"Out1\"],\"side\":\"RIGHT\"},\"type\":\"ConnectorPlacement.EquallySpacedRectSide\",\"uuid\":\"c83f4e01-5d94-498a-a9de-b4a302d500ab\"},{\"content\":{\"connectorIds\":[\"In3\"],\"side\":\"TOP\"},\"type\":\"ConnectorPlacement.EquallySpacedRectSide\",\"uuid\":\"3a6496e3-470c-4361-9f8f-cd28e1556398\"}]},\"type\":\"ConnectorPlacement.EquallySpacedConnector\",\"uuid\":\"b738ec8a-20ee-4a0a-8362-4988f331d970\"}],\"packageUris\":[\"http://schema.mathworks.com/mf0/Connector/R2020b\"],\"version\":\"1.0\"}"
  θ' : Subsystem  Priority=10  TreatAsAtomicUnit=on
      settings: PortSchema="{\"entries\":[{\"content\":{\"sides\":[{\"content\":{\"connectorIds\":[\"In1\"]},\"type\":\"ConnectorPlacement.EquallySpacedRectSide\",\"uuid\":\"9184f415-d771-478b-8114-38f854f6aad6\"},{\"content\":{\"connectorIds\":[\"Out1\"],\"side\":\"RIGHT\"},\"type\":\"ConnectorPlacement.EquallySpacedRectSide\",\"uuid\":\"399c2935-e635-4d1c-9ba7-451eea57bae3\"},{\"content\":{\"connectorIds\":[\"In2\"],\"side\":\"TOP\"},\"type\":\"ConnectorPlacement.EquallySpacedRectSide\",\"uuid\":\"bdc6ec05-8dca-4996-ba70-702aa29fd179\"}]},\"type\":\"ConnectorPlacement.EquallySpacedConnector\",\"uuid\":\"fa68c3f3-8285-4ee8-b99d-908dba81143c\"}],\"packageUris\":[\"http://schema.mathworks.com/mf0/Connector/R2020b\"],\"version\":\"1.0\"}"
  г(z) : Selector  InputPortWidth=2*dimension+1  IndexOptions=Index vector (dialog)  Indices=2:2:2*dimension  OutputSizes=1
  "∫θ " : Integrator  Priority=3  InitialCondition=initialTheta
  Ω out : Outport
  wires:
  Ф/1 -> Fu/1(Ф), Fc/3(Ф)
  y/1 -> Ω/2(y), Fu/5(y)
  z/1 -> г(z)/1, Fu/2(z), Fc/1(z)
  г(z)/1 -> Fc/4(Г(z)), Ω/3(г(z)), Fu/4(г(z))
  Ω in/1 -> Fc/2(Ω)
  ż/1 -> Fu/3(ż)
  "∫θ "/1 -> Ω/1(θ)
  Ω/1(Ω) -> Ω out/1
  Fc/1(Fc) -> θ'/2(Fc)
  Fu/1(Fu) -> θ'/1(Fu)
  θ'/1(θ') -> "∫θ "/1

== system adaptive_observer_for_sin_signal_original/Estimator mu=2.5/Subsystem ==
  Ω : Inport
  Constant1 : Constant  Value=r^2
  Divide : Product  Inputs=*/
  Gain1 : Gain  Gain=r^2
  Transpose{,1..3} (4 alike) : Math  Operator=transpose  SaturateOnIntegerOverflow=on
  Λ : Constant  Value=alpha
  Ω-Λ : Sum  Inputs=+-
  Ф : Outport
  wires:
  Divide/1 -> Ω-Λ/1
  Ω-Λ/1 -> Transpose1/1
  Ω/1 -> Divide/1
  Constant1/1 -> Divide/2
  Gain1/1 -> Transpose2/1
  Λ/1 -> Transpose/1
  Transpose/1 -> Gain1/1
  Transpose2/1 -> Ω-Λ/2
  Transpose1/1 -> Transpose3/1
  Transpose3/1 -> Ф/1

== system adaptive_observer_for_sin_signal_original/Estimator mu=2.5/Subsystem1 ==
  u : Inport
  Complex to Real-Imag : ComplexToRealImag
  MATLAB Function : MATLAB Function  TreatAsAtomicUnit=on
  Real-Imag to Complex : RealImagToComplex
  Switcher : Switch  Criteria=u2 ~= 0  Threshold=freqSwitcher(1)
  isComplex : Constant  Value=isComplex
  "∫Z " : Integrator  Priority=1  InitialCondition=real(initialZ)
  ∫Z 1 : Integrator  Priority=1  InitialCondition=imag(initialZ)
  Out1 : Outport
  wires:
  isComplex/1 -> Switcher/2
  u/1 -> MATLAB Function/1(zPrime), Complex to Real-Imag/1
  "∫Z "/1 -> Real-Imag to Complex/1, Switcher/1
  Switcher/1 -> Out1/1
  Complex to Real-Imag/1 -> "∫Z "/1
  Complex to Real-Imag/2 -> ∫Z 1/1
  ∫Z 1/1 -> Real-Imag to Complex/2
  Real-Imag to Complex/1 -> Switcher/3

== system adaptive_observer_for_sin_signal_original/Estimator mu=2.5/z' ==
  y : Inport
  Г(z) : Inport  Port=2
  Ф : Inport  Port=3
  z : Inport  Port=4
  Minus : Sum  Inputs=+-
  Product : Product  Multiplication=Matrix(*)
  S(z) : Subsystem
  Subsystem : Subsystem
  z' : Outport
  wires:
  z/1 -> Subsystem/4(z), S(z)/2(z)
  Minus/1 -> z'/1
  S(z)/1(S) -> Product/1
  Product/1 -> Minus/2
  Subsystem/1(zPreDot) -> Minus/1, Product/2, S(z)/1(zPreDot)
  Г(z)/1 -> Subsystem/1(bigGamma)
  Ф/1 -> Subsystem/2(PHI)
  y/1 -> Subsystem/3(y)

== system adaptive_observer_for_sin_signal_original/Estimator mu=5/Frequencies estimator ==
  Ф : Inport
  ż : Inport  Port=2
  Ω in : Inport  Port=3
  z : Inport  Port=4
  y : Inport  Port=5
  Fc : Subsystem  Priority=8  TreatAsAtomicUnit=on
      settings: PortSchema="{\"entries\":[{\"content\":{\"sides\":[{\"content\":{\"connectorIds\":[\"In1\",\"In2\",\"In3\"]},\"type\":\"ConnectorPlacement.EquallySpacedRectSide\",\"uuid\":\"ef8cffdc-1e6f-42c0-8cb3-bf318ca182f8\"},{\"content\":{\"connectorIds\":[\"Out1\"],\"side\":\"RIGHT\"},\"type\":\"ConnectorPlacement.EquallySpacedRectSide\",\"uuid\":\"a9c7e5b7-281a-47aa-808a-eb2877f3eee0\"},{\"content\":{\"connectorIds\":[\"In4\"],\"side\":\"TOP\"},\"type\":\"ConnectorPlacement.EquallySpacedRectSide\",\"uuid\":\"7bb4f6b5-7deb-4e08-9b2d-b96cfbb2c85e\"},{\"content\":{\"connectorIds\":[],\"side\":\"BOTTOM\"},\"type\":\"ConnectorPlacement.EquallySpacedRectSide\",\"uuid\":\"d628d464-6f95-4c60-8de5-a9188665a8a2\"}]},\"type\":\"ConnectorPlacement.EquallySpacedConnector\",\"uuid\":\"64fccc24-315d-40ff-920f-bd434d551c1a\"}],\"packageUris\":[\"http://schema.mathworks.com/mf0/Connector/R2020b\"],\"version\":\"1.0\"}"
  Fu : Subsystem  Priority=9  TreatAsAtomicUnit=on
      settings: PortSchema="{\"entries\":[{\"content\":{\"sides\":[{\"content\":{\"connectorIds\":[\"In1\",\"In2\"]},\"type\":\"ConnectorPlacement.EquallySpacedRectSide\",\"uuid\":\"56415c13-d553-4f88-94d3-75bcdc800e4b\"},{\"content\":{\"connectorIds\":[\"Out1\"],\"side\":\"RIGHT\"},\"type\":\"ConnectorPlacement.EquallySpacedRectSide\",\"uuid\":\"a1bdd2d2-4e49-40cb-b0b7-1df5316e4510\"},{\"content\":{\"connectorIds\":[\"In3\"],\"side\":\"TOP\"},\"type\":\"ConnectorPlacement.EquallySpacedRectSide\",\"uuid\":\"59b6ba3d-4a55-43e8-9b14-0d873cc3c9ca\"},{\"content\":{\"connectorIds\":[\"In4\",\"In5\"],\"side\":\"BOTTOM\"},\"type\":\"ConnectorPlacement.EquallySpacedRectSide\",\"uuid\":\"cb3db39e-f643-4fe7-a27f-76e86359c78d\"}]},\"type\":\"ConnectorPlacement.EquallySpacedConnector\",\"uuid\":\"fdf2e112-ecff-41aa-a5cb-d527a9dd51a8\"}],\"packageUris\":[\"http://schema.mathworks.com/mf0/Connector/R2020b\"],\"version\":\"1.0\"}"
  Ω : Subsystem  Priority=5  TreatAsAtomicUnit=on
      settings: PortSchema="{\"entries\":[{\"content\":{\"sides\":[{\"content\":{\"connectorIds\":[\"In1\",\"In2\"]},\"type\":\"ConnectorPlacement.EquallySpacedRectSide\",\"uuid\":\"0172ca52-64e8-432c-895c-e5829558e278\"},{\"content\":{\"connectorIds\":[\"Out1\"],\"side\":\"RIGHT\"},\"type\":\"ConnectorPlacement.EquallySpacedRectSide\",\"uuid\":\"c83f4e01-5d94-498a-a9de-b4a302d500ab\"},{\"content\":{\"connectorIds\":[\"In3\"],\"side\":\"TOP\"},\"type\":\"ConnectorPlacement.EquallySpacedRectSide\",\"uuid\":\"3a6496e3-470c-4361-9f8f-cd28e1556398\"}]},\"type\":\"ConnectorPlacement.EquallySpacedConnector\",\"uuid\":\"b738ec8a-20ee-4a0a-8362-4988f331d970\"}],\"packageUris\":[\"http://schema.mathworks.com/mf0/Connector/R2020b\"],\"version\":\"1.0\"}"
  θ' : Subsystem  Priority=10  TreatAsAtomicUnit=on
      settings: PortSchema="{\"entries\":[{\"content\":{\"sides\":[{\"content\":{\"connectorIds\":[\"In1\"]},\"type\":\"ConnectorPlacement.EquallySpacedRectSide\",\"uuid\":\"9184f415-d771-478b-8114-38f854f6aad6\"},{\"content\":{\"connectorIds\":[\"Out1\"],\"side\":\"RIGHT\"},\"type\":\"ConnectorPlacement.EquallySpacedRectSide\",\"uuid\":\"399c2935-e635-4d1c-9ba7-451eea57bae3\"},{\"content\":{\"connectorIds\":[\"In2\"],\"side\":\"TOP\"},\"type\":\"ConnectorPlacement.EquallySpacedRectSide\",\"uuid\":\"bdc6ec05-8dca-4996-ba70-702aa29fd179\"}]},\"type\":\"ConnectorPlacement.EquallySpacedConnector\",\"uuid\":\"fa68c3f3-8285-4ee8-b99d-908dba81143c\"}],\"packageUris\":[\"http://schema.mathworks.com/mf0/Connector/R2020b\"],\"version\":\"1.0\"}"
  г(z) : Selector  InputPortWidth=2*dimension+1  IndexOptions=Index vector (dialog)  Indices=2:2:2*dimension  OutputSizes=1
  "∫θ " : Integrator  Priority=3  InitialCondition=initialTheta
  Ω out : Outport
  wires:
  Ф/1 -> Fu/1(Ф), Fc/3(Ф)
  y/1 -> Ω/2(y), Fu/5(y)
  z/1 -> г(z)/1, Fu/2(z), Fc/1(z)
  г(z)/1 -> Fc/4(Г(z)), Ω/3(г(z)), Fu/4(г(z))
  Ω in/1 -> Fc/2(Ω)
  ż/1 -> Fu/3(ż)
  "∫θ "/1 -> Ω/1(θ)
  Ω/1(Ω) -> Ω out/1
  Fc/1(Fc) -> θ'/2(Fc)
  Fu/1(Fu) -> θ'/1(Fu)
  θ'/1(θ') -> "∫θ "/1

== system adaptive_observer_for_sin_signal_original/Estimator mu=5/Subsystem ==
  Ω : Inport
  Constant1 : Constant  Value=r^2
  Divide : Product  Inputs=*/
  Gain1 : Gain  Gain=r^2
  Transpose{,1..3} (4 alike) : Math  Operator=transpose  SaturateOnIntegerOverflow=on
  Λ : Constant  Value=alpha
  Ω-Λ : Sum  Inputs=+-
  Ф : Outport
  wires:
  Divide/1 -> Ω-Λ/1
  Ω-Λ/1 -> Transpose1/1
  Ω/1 -> Divide/1
  Constant1/1 -> Divide/2
  Gain1/1 -> Transpose2/1
  Λ/1 -> Transpose/1
  Transpose/1 -> Gain1/1
  Transpose2/1 -> Ω-Λ/2
  Transpose1/1 -> Transpose3/1
  Transpose3/1 -> Ф/1

== system adaptive_observer_for_sin_signal_original/Estimator mu=5/Subsystem1 ==
  u : Inport
  Complex to Real-Imag : ComplexToRealImag
  MATLAB Function : MATLAB Function  TreatAsAtomicUnit=on
  Real-Imag to Complex : RealImagToComplex
  Switcher : Switch  Criteria=u2 ~= 0  Threshold=freqSwitcher(1)
  isComplex : Constant  Value=isComplex
  "∫Z " : Integrator  Priority=1  InitialCondition=real(initialZ)
  ∫Z 1 : Integrator  Priority=1  InitialCondition=imag(initialZ)
  Out1 : Outport
  wires:
  isComplex/1 -> Switcher/2
  u/1 -> MATLAB Function/1(zPrime), Complex to Real-Imag/1
  "∫Z "/1 -> Real-Imag to Complex/1, Switcher/1
  Switcher/1 -> Out1/1
  Complex to Real-Imag/1 -> "∫Z "/1
  Complex to Real-Imag/2 -> ∫Z 1/1
  ∫Z 1/1 -> Real-Imag to Complex/2
  Real-Imag to Complex/1 -> Switcher/3

== system adaptive_observer_for_sin_signal_original/Estimator mu=5/z' ==
  y : Inport
  Г(z) : Inport  Port=2
  Ф : Inport  Port=3
  z : Inport  Port=4
  Minus : Sum  Inputs=+-
  Product : Product  Multiplication=Matrix(*)
  S(z) : Subsystem
  Subsystem : Subsystem
  z' : Outport
  wires:
  z/1 -> Subsystem/4(z), S(z)/2(z)
  Minus/1 -> z'/1
  S(z)/1(S) -> Product/1
  Product/1 -> Minus/2
  Subsystem/1(zPreDot) -> Minus/1, Product/2, S(z)/1(zPreDot)
  Г(z)/1 -> Subsystem/1(bigGamma)
  Ф/1 -> Subsystem/2(PHI)
  y/1 -> Subsystem/3(y)

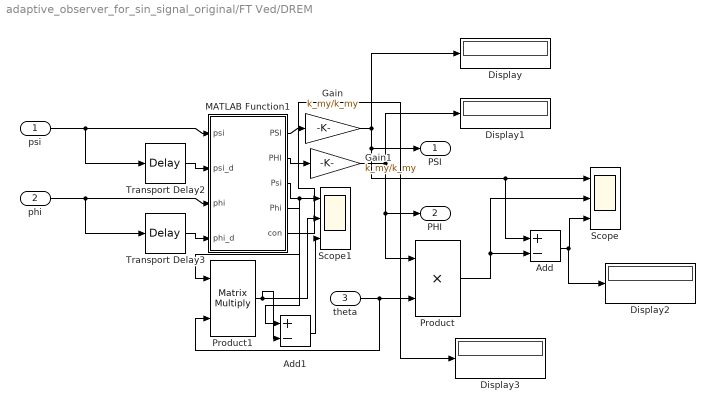
== system adaptive_observer_for_sin_signal_original/FT Ved/DREM ==
  psi : Inport
  phi : Inport  Port=2
  theta : Inport  Port=3
  Add : Sum  Inputs=+-
  Add1 : Sum  Inputs=+-
  Display{,1..3} (4 alike) : Display
  Gain : Gain  Gain=k_my/k_my
  Gain1 : Gain  Gain=k_my/k_my
  MATLAB Function1 : MATLAB Function  TreatAsAtomicUnit=on
  Product : Product
  Product1 : Product  Multiplication=Matrix(*)
  Scope : Scope  NumInputPorts=3
  Scope1 : Scope  NumInputPorts=3
  Transport Delay2 : TransportDelay  DelayTime=tau_my
  Transport Delay3 : TransportDelay  DelayTime=tau_my
  PSI : Outport  VectorParamsAs1DForOutWhenUnconnected=off
  PHI : Outport  Port=2  VectorParamsAs1DForOutWhenUnconnected=off
  wires:
  MATLAB Function1/1(PSI) -> Gain/1
  Transport Delay2/1 -> MATLAB Function1/2(psi_d)
  Transport Delay3/1 -> MATLAB Function1/4(phi_d)
  phi/1 -> Transport Delay3/1, MATLAB Function1/3(phi)
  psi/1 -> Transport Delay2/1, MATLAB Function1/1(psi)
  MATLAB Function1/2(PHI) -> Gain1/1
  Gain/1 -> Add/1, Scope/1, PSI/1, Display/1
  Gain1/1 -> Product/1, PHI/1, Display1/1
  Add/1 -> Display2/1, Scope/3
  Product/1 -> Scope/2, Add/2
  theta/1 -> Product1/2, Product/2
  MATLAB Function1/4(Phi) -> Product1/1
  MATLAB Function1/3(Psi) -> Scope1/1, Add1/1
  Product1/1 -> Add1/2, Scope1/2
  Add1/1 -> Scope1/3
  MATLAB Function1/5(con) -> Display3/1

== system adaptive_observer_for_sin_signal_original/FT Ved/Gradient1 ==
  note: \theta
  PSI : Inport
  PHI : Inport  Port=2
  Add1 : Sum  Inputs=+-
  Constant : Constant  Value=theta_real
  Divide2 : Product  Inputs=**
  Divide3 : Product  Inputs=**
  Gain1 : Gain  Gain=gamma_my
  Integrator1 : Integrator  InitialCondition=theta0_my
  MATLAB Function : MATLAB Function  TreatAsAtomicUnit=on
  Product : Product
  Product1 : Product
  Scope : Scope  NumInputPorts=3
  Scope1 : Scope
  Step : Step  Time=7*h_my+tau_my  SampleTime=0
  W : Subsystem
  theta_hat_ft : Outport  VectorParamsAs1DForOutWhenUnconnected=off
  wires:
  Gain1/1 -> Integrator1/1
  Divide3/1 -> Add1/2
  PSI/1 -> Product/2
  Step/1 -> Product1/1, Product/1
  Divide2/1 -> Gain1/1
  Add1/1 -> Divide2/2
  Integrator1/1 -> Scope/1, MATLAB Function/1(theta_hat), Divide3/2
  Product1/1 -> W/1(PHI), Divide2/1, Divide3/1
  Product/1 -> Add1/1
  PHI/1 -> Product1/2
  W/1(W) -> MATLAB Function/2(W), Scope1/1
  MATLAB Function/1(theta_ft) -> theta_hat_ft/1, Scope/2
  Constant/1 -> Scope/3

== system adaptive_observer_for_sin_signal_original/FT Ved/Regression model ==
  y : Inport
  Add : Sum  Inputs=+-
  MATLAB Function : MATLAB Function  TreatAsAtomicUnit=on
  Math Function : Math  Operator=transpose  SignedPower=on  SaturateOnIntegerOverflow=on
  Product : Product  Multiplication=Matrix(*)
  Scope : Scope  NumInputPorts=3
  Scope1 : Scope
  Transport Delay : TransportDelay  DelayTime=h_my
  Transport Delay1 : TransportDelay  DelayTime=2*h_my
  Transport Delay2 : TransportDelay  DelayTime=3*h_my
  Transport Delay3 : TransportDelay  DelayTime=4*h_my
  psi : Outport  VectorParamsAs1DForOutWhenUnconnected=off
  phi : Outport  Port=2  VectorParamsAs1DForOutWhenUnconnected=off
  theta : Outport  Port=3  VectorParamsAs1DForOutWhenUnconnected=off
  wires:
  y/1 -> MATLAB Function/1(y), Transport Delay/1, Transport Delay1/1, Transport Delay2/1, Transport Delay3/1
  Transport Delay/1 -> MATLAB Function/2(y1)
  Transport Delay1/1 -> MATLAB Function/3(y2)
  Transport Delay2/1 -> MATLAB Function/4(y3)
  Transport Delay3/1 -> MATLAB Function/5(y4)
  MATLAB Function/2(theta) -> theta/1, Math Function/1
  MATLAB Function/3(phi) -> phi/1, Product/2
  Product/1 -> Add/2, Scope/2
  Math Function/1 -> Product/1
  MATLAB Function/1(psi) -> Scope/1, Add/1, psi/1
  Add/1 -> Scope/3, Scope1/1

== system adaptive_observer_for_sin_signal_original/Original Signal/Source Signal ==
  Sum : Sum  Inputs=|++
  harmonic1 : Sin  Priority=0  Amplitude=amp(1)  Bias=bias(1)  Frequency=freq(1)  Phase=phase(1)  SampleTime=0
  harmonic2 : Sin  Priority=0  Amplitude=amp(2)  Bias=bias(2)  Frequency=freq(2)  Phase=phase(2)  SampleTime=0
  y : Outport
  wires:
  harmonic1/1 -> Sum/1
  harmonic2/1 -> Sum/2
  Sum/1 -> y/1

== system adaptive_observer_for_sin_signal_original/Original Signal/modifier ==
  y : Inport
  Band-Limited White Noise : simulink/Sources/Band-Limited White Noise  Cov=[0.00002]  Ts=0.001  seed=[23341]
  Sum : Sum  Inputs=|++
  Sum1 : Sum  Inputs=|++
  harmonic1 : Sin  Priority=0  Amplitude=amp_M1  Bias=bias_M1  Frequency=freq_M1  Phase=phase_M1  SampleTime=sample_M1
  harmonic3 : Sin  Priority=0  Amplitude=amp_M(1)  Bias=bias_M(1)  Frequency=freq_M(1)  Phase=phase_M(1)  SampleTime=0
  harmonic4 : Sin  Priority=0  Amplitude=amp_M(2)  Bias=bias_M(2)  Frequency=freq_M(2)  Phase=phase_M(2)  SampleTime=0
  noise or sin : Switch  Criteria=u2 > Threshold
  noise or sin? : Constant  Value=noiseOrSin
  switch or noise : Switch  Criteria=u2 > Threshold
  switch or noise? : Constant  Value=noiseOrSwitch
  y_mod : Outport
  wires:
  noise or sin?/1 -> noise or sin/2
  harmonic1/1 -> noise or sin/3
  Band-Limited White Noise/1 -> noise or sin/1
  harmonic3/1 -> Sum1/1
  harmonic4/1 -> Sum1/2
  switch or noise?/1 -> switch or noise/2
  Sum1/1 -> switch or noise/3
  y/1 -> Sum/2
  Sum/1 -> switch or noise/1
  noise or sin/1 -> Sum/1
  switch or noise/1 -> y_mod/1

== system adaptive_observer_for_sin_signal_original/Original Signal/mods enabler ==
  note: Время выключения внешних воздействий
  note: "1" - включить моды.
      | "0" - выключить моды
  note: Исходный сигнал
  Timer : Clock
  mods on? : Constant  Value=turn_mods_on
  mods turn on? : Switch  Criteria=u2 > Threshold
  timer mods off : Switch  Criteria=u2 > Threshold  Threshold=freqSwitcher(2)
  zero : Constant  Value=0
  zero1 : Constant  Value=0
  on_off : Outport
  wires:
  zero/1 -> mods turn on?/3
  mods on?/1 -> mods turn on?/2
  Timer/1 -> timer mods off/2, mods turn on?/1
  mods turn on?/1 -> timer mods off/3
  timer mods off/1 -> on_off/1
  zero1/1 -> timer mods off/1

== system adaptive_observer_for_sin_signal_original/Proposed Estimator/Frequencies estimator ==
  Ф : Inport
  ż : Inport  Port=2
  Ω in : Inport  Port=3
  z : Inport  Port=4
  y : Inport  Port=5
  Fc : Subsystem  Priority=8  TreatAsAtomicUnit=on
      settings: PortSchema="{\"entries\":[{\"content\":{\"sides\":[{\"content\":{\"connectorIds\":[\"In1\",\"In2\",\"In3\"]},\"type\":\"ConnectorPlacement.EquallySpacedRectSide\",\"uuid\":\"ef8cffdc-1e6f-42c0-8cb3-bf318ca182f8\"},{\"content\":{\"connectorIds\":[\"Out1\"],\"side\":\"RIGHT\"},\"type\":\"ConnectorPlacement.EquallySpacedRectSide\",\"uuid\":\"a9c7e5b7-281a-47aa-808a-eb2877f3eee0\"},{\"content\":{\"connectorIds\":[\"In4\"],\"side\":\"TOP\"},\"type\":\"ConnectorPlacement.EquallySpacedRectSide\",\"uuid\":\"7bb4f6b5-7deb-4e08-9b2d-b96cfbb2c85e\"},{\"content\":{\"connectorIds\":[],\"side\":\"BOTTOM\"},\"type\":\"ConnectorPlacement.EquallySpacedRectSide\",\"uuid\":\"d628d464-6f95-4c60-8de5-a9188665a8a2\"}]},\"type\":\"ConnectorPlacement.EquallySpacedConnector\",\"uuid\":\"64fccc24-315d-40ff-920f-bd434d551c1a\"}],\"packageUris\":[\"http://schema.mathworks.com/mf0/Connector/R2020b\"],\"version\":\"1.0\"}"
  Fu : Subsystem  Priority=9  TreatAsAtomicUnit=on
      settings: PortSchema="{\"entries\":[{\"content\":{\"sides\":[{\"content\":{\"connectorIds\":[\"In1\",\"In2\"]},\"type\":\"ConnectorPlacement.EquallySpacedRectSide\",\"uuid\":\"56415c13-d553-4f88-94d3-75bcdc800e4b\"},{\"content\":{\"connectorIds\":[\"Out1\"],\"side\":\"RIGHT\"},\"type\":\"ConnectorPlacement.EquallySpacedRectSide\",\"uuid\":\"a1bdd2d2-4e49-40cb-b0b7-1df5316e4510\"},{\"content\":{\"connectorIds\":[\"In3\"],\"side\":\"TOP\"},\"type\":\"ConnectorPlacement.EquallySpacedRectSide\",\"uuid\":\"59b6ba3d-4a55-43e8-9b14-0d873cc3c9ca\"},{\"content\":{\"connectorIds\":[\"In4\",\"In5\"],\"side\":\"BOTTOM\"},\"type\":\"ConnectorPlacement.EquallySpacedRectSide\",\"uuid\":\"cb3db39e-f643-4fe7-a27f-76e86359c78d\"}]},\"type\":\"ConnectorPlacement.EquallySpacedConnector\",\"uuid\":\"fdf2e112-ecff-41aa-a5cb-d527a9dd51a8\"}],\"packageUris\":[\"http://schema.mathworks.com/mf0/Connector/R2020b\"],\"version\":\"1.0\"}"
  Ω : Subsystem  Priority=5  TreatAsAtomicUnit=on
      settings: PortSchema="{\"entries\":[{\"content\":{\"sides\":[{\"content\":{\"connectorIds\":[\"In1\",\"In2\"]},\"type\":\"ConnectorPlacement.EquallySpacedRectSide\",\"uuid\":\"0172ca52-64e8-432c-895c-e5829558e278\"},{\"content\":{\"connectorIds\":[\"Out1\"],\"side\":\"RIGHT\"},\"type\":\"ConnectorPlacement.EquallySpacedRectSide\",\"uuid\":\"c83f4e01-5d94-498a-a9de-b4a302d500ab\"},{\"content\":{\"connectorIds\":[\"In3\"],\"side\":\"TOP\"},\"type\":\"ConnectorPlacement.EquallySpacedRectSide\",\"uuid\":\"3a6496e3-470c-4361-9f8f-cd28e1556398\"}]},\"type\":\"ConnectorPlacement.EquallySpacedConnector\",\"uuid\":\"b738ec8a-20ee-4a0a-8362-4988f331d970\"}],\"packageUris\":[\"http://schema.mathworks.com/mf0/Connector/R2020b\"],\"version\":\"1.0\"}"
  θ' : Subsystem  Priority=10  TreatAsAtomicUnit=on
      settings: PortSchema="{\"entries\":[{\"content\":{\"sides\":[{\"content\":{\"connectorIds\":[\"In1\"]},\"type\":\"ConnectorPlacement.EquallySpacedRectSide\",\"uuid\":\"9184f415-d771-478b-8114-38f854f6aad6\"},{\"content\":{\"connectorIds\":[\"Out1\"],\"side\":\"RIGHT\"},\"type\":\"ConnectorPlacement.EquallySpacedRectSide\",\"uuid\":\"399c2935-e635-4d1c-9ba7-451eea57bae3\"},{\"content\":{\"connectorIds\":[\"In2\"],\"side\":\"TOP\"},\"type\":\"ConnectorPlacement.EquallySpacedRectSide\",\"uuid\":\"bdc6ec05-8dca-4996-ba70-702aa29fd179\"}]},\"type\":\"ConnectorPlacement.EquallySpacedConnector\",\"uuid\":\"fa68c3f3-8285-4ee8-b99d-908dba81143c\"}],\"packageUris\":[\"http://schema.mathworks.com/mf0/Connector/R2020b\"],\"version\":\"1.0\"}"
  г(z) : Selector  InputPortWidth=2*dimension+1  IndexOptions=Index vector (dialog)  Indices=2:2:2*dimension  OutputSizes=1
  "∫θ " : Integrator  Priority=3  InitialCondition=initialTheta
  Ω out : Outport
  wires:
  Ф/1 -> Fu/1(Ф), Fc/3(Ф)
  y/1 -> Ω/2(y), Fu/5(y)
  z/1 -> г(z)/1, Fu/2(z), Fc/1(z)
  г(z)/1 -> Fc/4(Г(z)), Ω/3(г(z)), Fu/4(г(z))
  Ω in/1 -> Fc/2(Ω)
  ż/1 -> Fu/3(ż)
  "∫θ "/1 -> Ω/1(θ)
  Ω/1(Ω) -> Ω out/1
  Fc/1(Fc) -> θ'/2(Fc)
  Fu/1(Fu) -> θ'/1(Fu)
  θ'/1(θ') -> "∫θ "/1
